simulink model "simple_controller"  (R2023b)
settings: Solver=VariableStepAuto  StartTime=0.0  StopTime=50  RelTol=1e-3
undefined symbols (not defined in the file): dens, grav, m, vol
libraries: robotcorelib x1
settings Model: Creator=fabio  LastModifiedBy=fabio

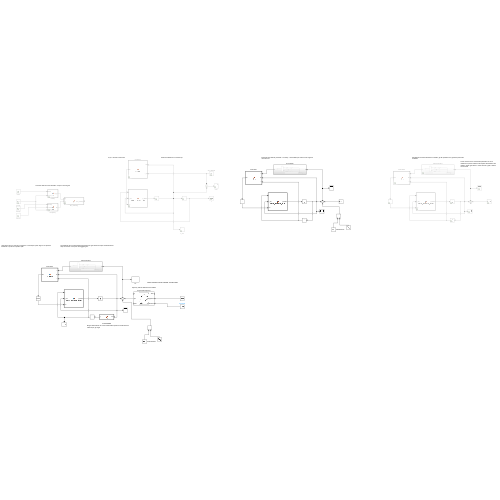
[thumbnail: Simulink's stored preview of the top-level diagram]
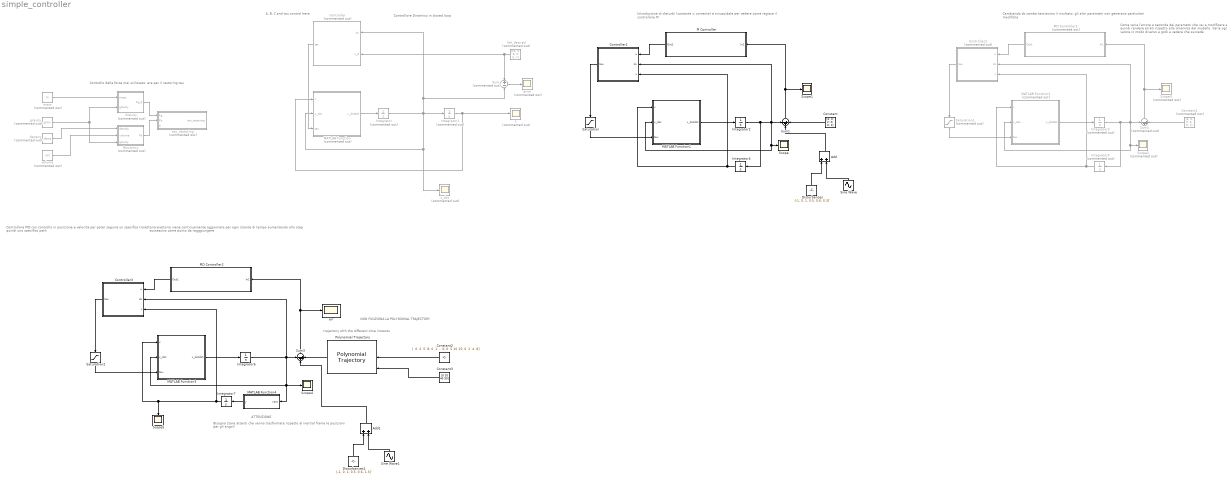
== system simple_controller ==
  note: NON FUNZIONA LA POLYNOMIAL TRAJECTORY
  note: Bisogna stare attenti che vanno trasformate rispetto al inertial frame le posizioni per gli angoli
  note: ATTENZIONE
  note: trajectory with the different time instants
  note: La traiettoria viene continuamente aggiornata per ogni istante di tempo aumentando allo step successivo come punto da ragggiungere
  note: Cambiando zb camba tantissimo il risultato, gli altri paramteri non generano particolari modifiche
  note: Controllore PID con controllo in posizione e velocità per poter seguire un specifica traiettoria e quindi uno specifico path
  note: Controllo delle forze mai utilizzato. era per il restoring tau
  note: Controllore Dinamico in closed loop
  note: Introduzione di disturbi (costante = corrente) e sinusoidale per vedere come regisce il controllore PI
  note: Come varia l'errore a seconda dei parametri che vai a modificare e quindi rendere errati rispetto alla dinamica del modello. Varia ogni valore in modo diverso e godi a vedere che succede
  note: A, B, C and tau control here
  Add : Sum
  Add1 : Sum
  Bouyancy : MATLAB Function  Commented=on  TreatAsAtomicUnit=on
  Constant : Constant  Value=[3; 0; 2; 0; 0; 1]
  Constant1 : Constant  Commented=on  Value=[3; 0; 2; 0; 0; 1]
  Constant2 : Constant  Value="[  0  2  5  8; 0  1  3  6; 0  0  1  2;  0  0 0 0; 0  5 10 15; 0  2  4  8]"
  Constant3 : Constant  Value=[0 20 40 50]
  Controller : MATLAB Function  Commented=on  TreatAsAtomicUnit=on
  Controller1 : MATLAB Function  TreatAsAtomicUnit=on
  Controller2 : MATLAB Function  Commented=on  TreatAsAtomicUnit=on
  Controller3 : MATLAB Function  TreatAsAtomicUnit=on
  Disturbances : Constant  Value=[-1, 0, 1, 0.5, 0.6, 0.3]'
  Disturbances1 : Constant  Value=[-1, 0, 1, 0.5, 0.6, 1.3]'
  Gravity : MATLAB Function  Commented=on  TreatAsAtomicUnit=on
  Integrator{,1,3,5} (4 alike) : Integrator  Commented=on
  Integrator{2,4,6..7} (4 alike) : Integrator
  MATLAB Function : MATLAB Function  Commented=on  TreatAsAtomicUnit=on
  MATLAB Function1 : MATLAB Function  TreatAsAtomicUnit=on
  MATLAB Function2 : MATLAB Function  Commented=on  TreatAsAtomicUnit=on
  MATLAB Function3 : MATLAB Function  TreatAsAtomicUnit=on
  MATLAB Function4 : MATLAB Function  TreatAsAtomicUnit=on
  PI Controller : Subsystem
  PID Controller1 : Subsystem  Commented=on
  PID Controller2 : Subsystem
  Polynomial Trajectory : robotcorelib/Polynomial Trajectory  WaypointSource=External  Waypoints="[  0  2  5  8; 0  1  3  6; 0  0  1  2;  0  0 0 0; 0  5 10 15; 0  2  4  8]"  TimePoints=[0 2 4 6]  TimeInterval=[ 1, 4 ]  Method=Quintic Polynomial  ParameterSource=Internal  VelocityBoundaryCondition=zeros(6,4)  AccelerationBoundaryCondition=zeros(6,4 )  SimulateUsing=Interpreted execution
  Saturation : Saturate  UpperLimit=20000  LowerLimit=-20000
  Saturation1 : Saturate  Commented=on  UpperLimit=20000  LowerLimit=-20000
  Saturation2 : Saturate  UpperLimit=20000  LowerLimit=-20000
  Scope{,1,4..5} (4 alike) : Scope
  Scope2 : Scope  Commented=on
  Scope3 : Scope  Commented=on
  Sine Wave : Sin  Amplitude=0.1  Frequency=0.05  SampleTime=0
  Sine Wave1 : Sin  Amplitude=0.5  Frequency=0.05  SampleTime=0
  Sum : Sum  Commented=on  Inputs=+-
  Sum1 : Sum  Inputs=-++
  Sum2 : Sum  Commented=on  Inputs=-++
  Sum3 : Sum  Inputs=-++
  Vel_desired : Constant  Commented=on  Value=[10; 0; 9; 0; 0; 7]
  density : Constant  Commented=on  Value=dens
  err : Scope
  error : Scope  Commented=on
  gravity : Constant  Commented=on  Value=grav
  mass : Constant  Commented=on  Value=m
  tau_restoring : MATLAB Function  Commented=on  TreatAsAtomicUnit=on
  volume : Constant  Commented=on  Value=vol
  x : Scope  Commented=on
  x_dot : Scope  Commented=on
  wires:
  MATLAB Function/1(x_dotdot) -> Integrator/1
  Integrator/1 -> Controller/1(dx), Sum/2, MATLAB Function/2(x_dot), x_dot/1, Integrator1/1
  Integrator1/1 -> MATLAB Function/1(x), x/1
  gravity/1 -> Bouyancy/3(gravity), Gravity/2(gravity)
  volume/1 -> Bouyancy/2(volume)
  density/1 -> Bouyancy/1(density)
  mass/1 -> Gravity/1(mass)
  Gravity/1(Fg_b) -> tau_restoring/1(Fg)
  Bouyancy/1(Fb) -> tau_restoring/2(Fb)
  Vel_desired/1 -> Sum/1, Controller/2(v_d)
  Sum/1 -> error/1
  Controller/1(tau) -> MATLAB Function/3(tau)
  MATLAB Function1/1(x_dotdot) -> Integrator2/1
  Integrator2/1 -> Integrator4/1, MATLAB Function1/2(x_dot), Scope/1, Controller1/2(dx), Sum1/1
  Integrator4/1 -> Controller1/3(x), MATLAB Function1/1(x)
  Sum1/1 -> PI Controller/1(In1), Scope1/1
  PI Controller/1(Out1) -> Controller1/1(u)
  Constant/1 -> Sum1/3
  Controller1/1(tau) -> Saturation/1
  Saturation/1 -> MATLAB Function1/3(tau)
  Add/1 -> Sum1/2
  Disturbances/1 -> Add/1
  Sine Wave/1 -> Add/2
  Constant1/1 -> Sum2/3
  Saturation1/1 -> MATLAB Function2/3(tau)
  Integrator3/1 -> Integrator5/1, MATLAB Function2/2(x_dot), Scope2/1, Controller2/2(dx), Sum2/1
  Sum2/1 -> PID Controller1/1(In1), Scope3/1
  Controller2/1(tau) -> Saturation1/1
  MATLAB Function2/1(x_dotdot) -> Integrator3/1
  PID Controller1/1(Out1) -> Controller2/1(u)
  Integrator5/1 -> Controller2/3(x), MATLAB Function2/1(x)
  Saturation2/1 -> MATLAB Function3/3(tau)
  Integrator6/1 -> MATLAB Function4/1(vect), MATLAB Function3/2(x_dot), Scope4/1, Controller3/2(dx), Sum3/1
  PID Controller2/1(Out1) -> Controller3/1(u)
  MATLAB Function3/1(x_dotdot) -> Integrator6/1
  Integrator7/1 -> Controller3/3(x), MATLAB Function3/1(x), Scope5/1
  Controller3/1(tau) -> Saturation2/1
  Sum3/1 -> PID Controller2/1(In1), err/1
  Add1/1 -> Sum3/2
  Disturbances1/1 -> Add1/1
  Sine Wave1/1 -> Add1/2
  MATLAB Function4/1(y) -> Integrator7/1
  Polynomial Trajectory/2 -> Sum3/3
  Constant2/1 -> Polynomial Trajectory/2
  Constant3/1 -> Polynomial Trajectory/3

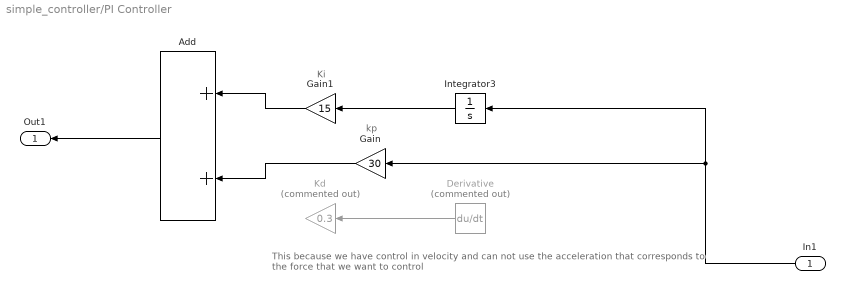
== system simple_controller/PI Controller ==
  note: This because we have control in velocity and can not use the acceleration that corresponds to the force that we want to control
  note: Ki
  note: kp
  In1 : Inport
  Add : Sum
  Derivative : Derivative  Commented=on
  Gain : Gain  Gain=30
  Gain1 : Gain  Gain=15
  Integrator3 : Integrator
  Kd : Gain  Commented=on  Gain=0.3
  Out1 : Outport
  wires:
  Derivative/1 -> Kd/1
  Gain/1 -> Add/2
  Integrator3/1 -> Gain1/1
  In1/1 -> Integrator3/1, Gain/1
  Add/1 -> Out1/1
  Gain1/1 -> Add/1

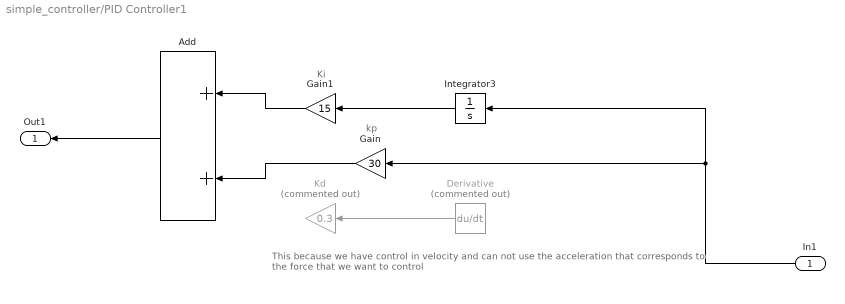
== system simple_controller/PID Controller1 ==
  note: This because we have control in velocity and can not use the acceleration that corresponds to the force that we want to control
  note: Ki
  note: kp
  In1 : Inport
  Add : Sum
  Derivative : Derivative  Commented=on
  Gain : Gain  Gain=30
  Gain1 : Gain  Gain=15
  Integrator3 : Integrator
  Kd : Gain  Commented=on  Gain=0.3
  Out1 : Outport
  wires:
  Derivative/1 -> Kd/1
  Gain/1 -> Add/2
  Integrator3/1 -> Gain1/1
  In1/1 -> Integrator3/1, Gain/1
  Add/1 -> Out1/1
  Gain1/1 -> Add/1

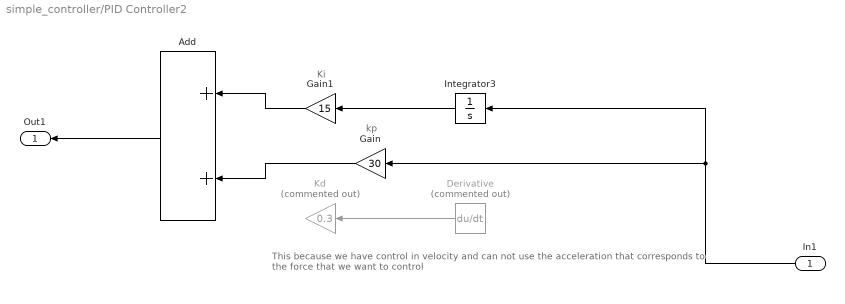
== system simple_controller/PID Controller2 ==
  note: This because we have control in velocity and can not use the acceleration that corresponds to the force that we want to control
  note: Ki
  note: kp
  In1 : Inport
  Add : Sum
  Derivative : Derivative  Commented=on
  Gain : Gain  Gain=30
  Gain1 : Gain  Gain=15
  Integrator3 : Integrator
  Kd : Gain  Commented=on  Gain=0.3
  Out1 : Outport
  wires:
  Derivative/1 -> Kd/1
  Gain/1 -> Add/2
  Integrator3/1 -> Gain1/1
  In1/1 -> Integrator3/1, Gain/1
  Add/1 -> Out1/1
  Gain1/1 -> Add/1

== matlab function simple_controller/MATLAB Function3 ==
  data: x input; x_dot input; tau input; x_dotdot output
function x_dotdot = vehicle_dynamics_matrix(x, x_dot, tau)
    m = 4000;
    B = 39200;
    I = diag([2507, 1367, 2660]);
    zb = -0.36;

    % Added mass
    tau_a = [-290; -310; -535; -89; -137; -95];

    % Restoring forces
    tau_r = [-360; -420; -400; -60; -130; -110];

    % Hydrodynamic forces
    tau_d = [-805; -1930; -1650; -304; -658; -555];

    % Virtual mass
    mv = [m; m; m; I(1,1); I(2,2); I(3,3)] - tau_a;

    % Dissatipative forces
    dv = -tau_r - tau_d .* abs(x_dot);

    % Accelerations
    x_dotdot = zeros(6,1);
    
    x_dotdot(1) = (tau(1) + mv(2)*x_dot(2)*x_dot(6) - mv(3)*x_dot(3)*x_dot(5) - dv(1)*x_dot(1)) / mv(1); 
    x_dotdot(2) = (tau(2) - mv(1)*x_dot(1)*x_dot(6) + mv(3)*x_dot(3)*x_dot(4) - dv(2)*x_dot(2)) / mv(2);
    x_dotdot(3) = (tau(3) + mv(1)*x_dot(1)*x_dot(5) - mv(2)*x_dot(2)*x_dot(4) - dv(3)*x_dot(3)) / mv(3);
    x_dotdot(4) = (tau(4) + (mv(2) - mv(3))*x_dot(2)*x_dot(3) + (mv(5) - mv(6))*x_dot(5)*x_dot(6) - dv(4)*x_dot(4) - zb*B*cos(x(5))*sin(x(4))) / mv(4);
    x_dotdot(5) = (tau(5) - (mv(1) - mv(3))*x_dot(1)*x_dot(3) - (mv(4) - mv(6))*x_dot(4)*x_dot(6) - dv(5)*x_dot(5) + zb*B*sin(x(5))) / mv(5);
    x_dotdot(6) = (tau(6) + (mv(1) - mv(2))*x_dot(1)*x_dot(2) + (mv(4) - mv(5))*x_dot(4)*x_dot(5) - dv(6)*x_dot(6)) / mv(6);
end

== matlab function simple_controller/MATLAB Function4 ==
  data: y output; vect input
function y = mapping(vect)
    % Transformation from body farme to inertial frame of velocities
    p = vect(4:6);
    Jacobian = zeros(6,6);
    Jacobian(1:3, 1:3) = [cos(p(3))*cos(p(2)), -sin(p(3))*cos(p(1))+cos(p(3))*sin(p(2))*sin(p(1)), sin(p(3))*sin(p(1))+cos(p(3))*sin(p(2))*cos(p(1)); ...
                    sin(p(3))*cos(p(2)), cos(p(3))*cos(p(1))+sin(p(3))*sin(p(2))*sin(p(1)), -cos(p(3))*sin(p(2))*cos(p(1)); ...
                    -sin(p(2)), cos(p(2))*sin(p(1)), cos(p(2))*cos(p(1))];
    Jacobian(4:6, 4:6) = [1, sin(p(1))*tan(p(2)), cos(p(1))*tan(p(2));
                        0, cos(p(1)), -sin(p(1));
                        0, sin(p(1))/cos(p(2)), cos(p(1))/cos(p(2))];
    y = Jacobian * vect;
end

== matlab function simple_controller/Gravity ==
  data: mass input; Fg_b output; gravity input
function Fg_b = fcn(mass, gravity)
    Fg = mass * gravity;
    p = pos(4:6);
    rotation = [cos(p(3))*cos(p(2)), -sin(p(3))*cos(p(1))+cos(p(3))*sin(p(2))*sin(p(1)), sin(p(3))*sin(p(1))+cos(p(3))*sin(p(2))*cos(p(1)); ...
                sin(p(3))*cos(p(2)), cos(p(3))*cos(p(1))+sin(p(3))*sin(p(2))*sin(p(1)), -cos(p(3))*sin(p(2))*cos(p(1)); ...
                -sin(p(2)), cos(p(2))*sin(p(1)), cos(p(2))*cos(p(1))];
    Fg_b = (rotation)' * Fg;
end

== matlab function simple_controller/MATLAB Function ==
  data: x input; x_dot input; tau input; x_dotdot output
function x_dotdot = vehicle_dynamics_matrix(x, x_dot, tau)
    m = 4000;
    B = 39200;
    I = diag([2507, 1367, 2660]);
    zb = -0.36;

    % Added mass
    tau_a = [-290; -310; -535; -89; -137; -95];

    % Restoring forces
    tau_r = [-360; -420; -400; -60; -130; -110];

    % Hydrodynamic forces
    tau_d = [-805; -1930; -1650; -304; -658; -555];

    % Virtual mass
    mv = [m; m; m; I(1,1); I(2,2); I(3,3)] - tau_a;

    % Dissatipative forces
    dv = -tau_r - tau_d .* abs(x_dot);

    % Accelerations
    x_dotdot = zeros(6,1);
    
    x_dotdot(1) = (tau(1) + mv(2)*x_dot(2)*x_dot(6) - mv(3)*x_dot(3)*x_dot(5) - dv(1)*x_dot(1)) / mv(1); 
    x_dotdot(2) = (tau(2) - mv(1)*x_dot(1)*x_dot(6) + mv(3)*x_dot(3)*x_dot(4) - dv(2)*x_dot(2)) / mv(2);
    x_dotdot(3) = (tau(3) + mv(1)*x_dot(1)*x_dot(5) - mv(2)*x_dot(2)*x_dot(4) - dv(3)*x_dot(3)) / mv(3);
    x_dotdot(4) = (tau(4) + (mv(2) - mv(3))*x_dot(2)*x_dot(3) + (mv(5) - mv(6))*x_dot(5)*x_dot(6) - dv(4)*x_dot(4) - zb*B*cos(x(5))*sin(x(4))) / mv(4);
    x_dotdot(5) = (tau(5) - (mv(1) - mv(3))*x_dot(1)*x_dot(3) - (mv(4) - mv(6))*x_dot(4)*x_dot(6) - dv(5)*x_dot(5) + zb*B*sin(x(5))) / mv(5);
    x_dotdot(6) = (tau(6) + (mv(1) - mv(2))*x_dot(1)*x_dot(2) + (mv(4) - mv(5))*x_dot(4)*x_dot(5) - dv(6)*x_dot(6)) / mv(6);
end

== matlab function simple_controller/Bouyancy ==
  data: density input; Fb output; volume input; gravity input
function Fb = fcn(density, volume, gravity)
    Fb = volume * density * gravity;
end

== matlab function simple_controller/tau_restoring ==
  data: Fg input; tau_restoring output; Fb input; p input
function tau_restoring = fcn(Fg, Fb, p)
    % Already the tau needed
    tau_restoring = ((rotation)' * Fg) - Fb;
end

== matlab function simple_controller/Controller ==
  data: dx input; v_d input; tau output
function tau = controller(dx, v_d)
    m = 4000;
    B = 39200;
    err = v_d - dx;
    K = 1000;
    zb = -0.36;
    I = diag([2507, 1367, 2660]);

    % Added mass
    tau_a = [-290; -310; -535; -89; -137; -95];

    % Restoring forces
    tau_r = [-360; -420; -400; -60; -130; -110];

    % Hydrodynamic forces
    tau_d = [-805; -1930; -1650; -304; -658; -555];

    % Virtual mass
    mv = [m; m; m; I(1,1); I(2,2); I(3,3)] - tau_a;

    % Dissatipative forces
    dv = -tau_r - tau_d .* abs(dx);

    tau = zeros(6,1);
    tau(1) = mv(1)*K*err(1) - mv(2)*dx(2)*dx(6) + mv(3)*dx(3)*dx(5) + dv(1)*dx(1);
    % tau(2) = mv(2)*K*err(2) + mv(2)*dx(1)*dx(6) - mv(3)*dx(3)*dx(4) + dv(2)*dx(2);
    tau(3) = mv(3)*K*err(3) - mv(1)*dx(1)*dx(5) + mv(2)*dx(2)*dx(4) + dv(3)*dx(3);
    % tau(4) = mv(4)*K*err(4) - (mv(2) - mv(3))*dx(2)*dx(3) - (mv(5) - mv(6))*dx(5)*dx(6) + dv(4)*dx(4) + zb*B*cos(x(5))*sin(x(4));
    % tau(5) = mv(5)*K*err(5) + (mv(1) - mv(3))*dx(1)*dx(3) + (mv(4) - mv(6))*dx(4)*dx(6) + dv(5)*dx(5) - zb*B*sin(x(5));
    tau(6) = mv(6)*K*err(6) - (mv(1) - mv(2))*dx(1)*dx(2) - (mv(4) - mv(5))*dx(4)*dx(5) + dv(6)*dx(6);
end

== matlab function simple_controller/MATLAB Function1 ==
  data: x input; x_dot input; tau input; x_dotdot output
function x_dotdot = vehicle_dynamics_matrix(x, x_dot, tau)
    m = 4000;
    B = 39200;
    I = diag([2507, 1367, 2660]);
    zb = -0.36;

    % Added mass
    tau_a = [-290; -310; -535; -89; -137; -95];

    % Restoring forces
    tau_r = [-360; -420; -400; -60; -130; -110];

    % Hydrodynamic forces
    tau_d = [-805; -1930; -1650; -304; -658; -555];

    % Virtual mass
    mv = [m; m; m; I(1,1); I(2,2); I(3,3)] - tau_a;

    % Dissatipative forces
    dv = -tau_r - tau_d .* abs(x_dot);

    % Accelerations
    x_dotdot = zeros(6,1);
    
    x_dotdot(1) = (tau(1) + mv(2)*x_dot(2)*x_dot(6) - mv(3)*x_dot(3)*x_dot(5) - dv(1)*x_dot(1)) / mv(1); 
    x_dotdot(2) = (tau(2) - mv(1)*x_dot(1)*x_dot(6) + mv(3)*x_dot(3)*x_dot(4) - dv(2)*x_dot(2)) / mv(2);
    x_dotdot(3) = (tau(3) + mv(1)*x_dot(1)*x_dot(5) - mv(2)*x_dot(2)*x_dot(4) - dv(3)*x_dot(3)) / mv(3);
    x_dotdot(4) = (tau(4) + (mv(2) - mv(3))*x_dot(2)*x_dot(3) + (mv(5) - mv(6))*x_dot(5)*x_dot(6) - dv(4)*x_dot(4) - zb*B*cos(x(5))*sin(x(4))) / mv(4);
    x_dotdot(5) = (tau(5) - (mv(1) - mv(3))*x_dot(1)*x_dot(3) - (mv(4) - mv(6))*x_dot(4)*x_dot(6) - dv(5)*x_dot(5) + zb*B*sin(x(5))) / mv(5);
    x_dotdot(6) = (tau(6) + (mv(1) - mv(2))*x_dot(1)*x_dot(2) + (mv(4) - mv(5))*x_dot(4)*x_dot(5) - dv(6)*x_dot(6)) / mv(6);
end

== matlab function simple_controller/Controller1 ==
  data: u input; dx input; tau output; x input
function tau = controller(u, dx, x)
    m = 4000;
    B = 39200;
    K = 1;
    zb = -0.36;
    I = diag([2507, 1367, 2660]);

    % Added mass
    tau_a = [-290; -310; -535; -89; -137; -95];

    % Restoring forces
    tau_r = [-360; -420; -400; -60; -130; -110];

    % Hydrodynamic forces
    tau_d = [-805; -1930; -1650; -304; -658; -555];

    % Virtual mass
    mv = [m; m; m; I(1,1); I(2,2); I(3,3)] - tau_a;

    % Dissatipative forces
    dv = -tau_r - tau_d .* abs(dx);

    tau = zeros(6,1);
    tau(1) = mv(1)*K*u(1) - mv(2)*dx(2)*dx(6) + mv(3)*dx(3)*dx(5) + dv(1)*dx(1);
    % tau(2) = mv(2)*K*u(2) + mv(2)*dx(1)*dx(6) - mv(3)*dx(3)*dx(4) + dv(2)*dx(2);
    tau(3) = mv(3)*K*u(3) - mv(1)*dx(1)*dx(5) + mv(2)*dx(2)*dx(4) + dv(3)*dx(3);
    tau(4) = mv(4)*K*u(4) - (mv(2) - mv(3))*dx(2)*dx(3) - (mv(5) - mv(6))*dx(5)*dx(6) + dv(4)*dx(4) + zb*B*cos(x(5))*sin(x(4));
    tau(5) = mv(5)*K*u(5) + (mv(1) - mv(3))*dx(1)*dx(3) + (mv(4) - mv(6))*dx(4)*dx(6) + dv(5)*dx(5) - zb*B*sin(x(5));
    tau(6) = mv(6)*K*u(6) - (mv(1) - mv(2))*dx(1)*dx(2) - (mv(4) - mv(5))*dx(4)*dx(5) + dv(6)*dx(6);
end

== matlab function simple_controller/Controller2 ==
  data: u input; dx input; tau output; x input
function tau = controller(u, dx, x)
    m = 4200;
    B = 39000;
    K = 1;
    zb = -0.36;
    I = diag([2507, 1367, 2660]);

    % Added mass
    tau_a = [-300; -310; -535; -200; -137; -95];

    % Restoring forces
    tau_r = [-360; -420; -400; -60; -130; -110];

    % Hydrodynamic forces
    tau_d = [-805; -1930; -1650; -500; -658; -555];

    % Virtual mass
    mv = [m; m; m; I(1,1); I(2,2); I(3,3)] - tau_a;

    % Dissatipative forces
    dv = -tau_r - tau_d .* abs(dx);

    tau = zeros(6,1);
    tau(1) = mv(1)*K*u(1) - mv(2)*dx(2)*dx(6) + mv(3)*dx(3)*dx(5) + dv(1)*dx(1);
    %tau(2) = mv(2)*K*u(2) + mv(2)*dx(1)*dx(6) - mv(3)*dx(3)*dx(4) + dv(2)*dx(2);
    tau(3) = mv(3)*K*u(3) - mv(1)*dx(1)*dx(5) + mv(2)*dx(2)*dx(4) + dv(3)*dx(3);
    tau(4) = mv(4)*K*u(4) - (mv(2) - mv(3))*dx(2)*dx(3) - (mv(5) - mv(6))*dx(5)*dx(6) + dv(4)*dx(4) + zb*B*cos(x(5))*sin(x(4));
    tau(5) = mv(5)*K*u(5) + (mv(1) - mv(3))*dx(1)*dx(3) + (mv(4) - mv(6))*dx(4)*dx(6) + dv(5)*dx(5) - zb*B*sin(x(5));
    tau(6) = mv(6)*K*u(6) - (mv(1) - mv(2))*dx(1)*dx(2) - (mv(4) - mv(5))*dx(4)*dx(5) + dv(6)*dx(6);
end

== matlab function simple_controller/MATLAB Function2 ==
  data: x input; x_dot input; tau input; x_dotdot output
function x_dotdot = vehicle_dynamics_matrix(x, x_dot, tau)
    m = 4000;
    B = 39200;
    I = diag([2507, 1367, 2660]);
    zb = -0.36;

    % Added mass
    tau_a = [-290; -310; -535; -89; -137; -95];

    % Restoring forces
    tau_r = [-360; -420; -400; -60; -130; -110];

    % Hydrodynamic forces
    tau_d = [-805; -1930; -1650; -304; -658; -555];

    % Virtual mass
    mv = [m; m; m; I(1,1); I(2,2); I(3,3)] - tau_a;

    % Dissatipative forces
    dv = -tau_r - tau_d .* abs(x_dot);

    % Accelerations
    x_dotdot = zeros(6,1);
    
    x_dotdot(1) = (tau(1) + mv(2)*x_dot(2)*x_dot(6) - mv(3)*x_dot(3)*x_dot(5) - dv(1)*x_dot(1)) / mv(1); 
    x_dotdot(2) = (tau(2) - mv(1)*x_dot(1)*x_dot(6) + mv(3)*x_dot(3)*x_dot(4) - dv(2)*x_dot(2)) / mv(2);
    x_dotdot(3) = (tau(3) + mv(1)*x_dot(1)*x_dot(5) - mv(2)*x_dot(2)*x_dot(4) - dv(3)*x_dot(3)) / mv(3);
    x_dotdot(4) = (tau(4) + (mv(2) - mv(3))*x_dot(2)*x_dot(3) + (mv(5) - mv(6))*x_dot(5)*x_dot(6) - dv(4)*x_dot(4) - zb*B*cos(x(5))*sin(x(4))) / mv(4);
    x_dotdot(5) = (tau(5) - (mv(1) - mv(3))*x_dot(1)*x_dot(3) - (mv(4) - mv(6))*x_dot(4)*x_dot(6) - dv(5)*x_dot(5) + zb*B*sin(x(5))) / mv(5);
    x_dotdot(6) = (tau(6) + (mv(1) - mv(2))*x_dot(1)*x_dot(2) + (mv(4) - mv(5))*x_dot(4)*x_dot(5) - dv(6)*x_dot(6)) / mv(6);
end

== matlab function simple_controller/Controller3 ==
  data: u input; dx input; tau output; x input
function tau = controller(u, dx, x)
    m = 4200;
    B = 39000;
    K = 1;
    zb = -0.36;
    I = diag([2507, 1367, 2660]);

    % Added mass
    tau_a = [-300; -310; -535; -200; -137; -95];

    % Restoring forces
    tau_r = [-360; -420; -400; -60; -130; -110];

    % Hydrodynamic forces
    tau_d = [-805; -1930; -1650; -500; -658; -555];

    % Virtual mass
    mv = [m; m; m; I(1,1); I(2,2); I(3,3)] - tau_a;

    % Dissatipative forces
    dv = -tau_r - tau_d .* abs(dx);

    tau = zeros(6,1);
    tau(1) = mv(1)*K*u(1) - mv(2)*dx(2)*dx(6) + mv(3)*dx(3)*dx(5) + dv(1)*dx(1);
    %tau(2) = mv(2)*K*u(2) + mv(2)*dx(1)*dx(6) - mv(3)*dx(3)*dx(4) + dv(2)*dx(2);
    tau(3) = mv(3)*K*u(3) - mv(1)*dx(1)*dx(5) + mv(2)*dx(2)*dx(4) + dv(3)*dx(3);
    tau(4) = mv(4)*K*u(4) - (mv(2) - mv(3))*dx(2)*dx(3) - (mv(5) - mv(6))*dx(5)*dx(6) + dv(4)*dx(4) + zb*B*cos(x(5))*sin(x(4));
    tau(5) = mv(5)*K*u(5) + (mv(1) - mv(3))*dx(1)*dx(3) + (mv(4) - mv(6))*dx(4)*dx(6) + dv(5)*dx(5) - zb*B*sin(x(5));
    tau(6) = mv(6)*K*u(6) - (mv(1) - mv(2))*dx(1)*dx(2) - (mv(4) - mv(5))*dx(4)*dx(5) + dv(6)*dx(6);
end
